simulink model "Simulink_Problema2_2"  (R2020b)
settings: Solver=VariableStepAuto  StartTime=0.0  StopTime=10.0  RelTol=1e-3
libraries: dsparch4 x2
settings Model: Creator=enrique  LastModifiedBy=enrique

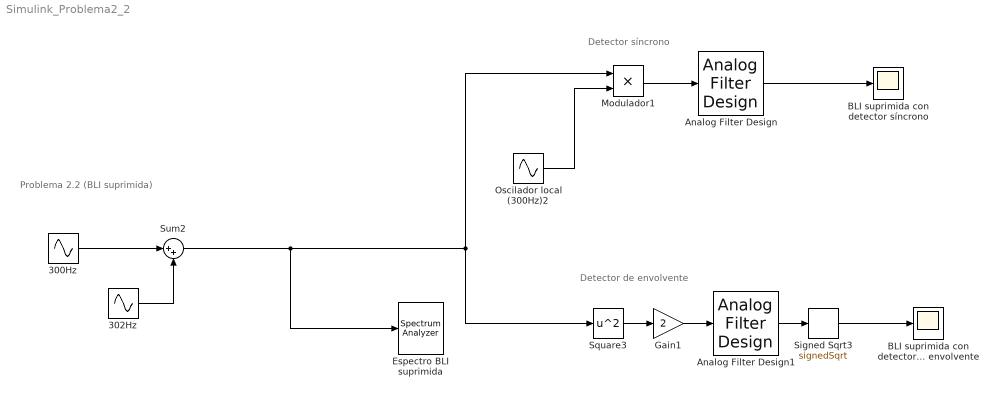
== system Simulink_Problema2_2 ==
  note: Problema 2.2 (BLI suprimida)
  note: Detector síncrono
  note: Detector de envolvente
  300Hz : Sin  Frequency=2*pi*300  SampleTime=1/5000
  302Hz : Sin  Amplitude=0.8  Frequency=2*pi*302  SampleTime=1/5000
  Analog Filter Design : dsparch4/Analog Filter Design  method=Butterworth  filttype=Lowpass  N=4  Wlo=2*pi*10  Whi=80  Rp=2  Rs=40
  Analog Filter Design1 : dsparch4/Analog Filter Design  method=Butterworth  filttype=Lowpass  N=4  Wlo=2*pi*10  Whi=80  Rp=2  Rs=40
  BLI suprimida con detector síncrono : Scope
  BLI suprimida con detector de envolvente : Scope
  Espectro BLI suprimida : SpectrumAnalyzer
  Gain1 : Gain  Gain=2
  Modulador1 : Product  OutDataTypeStr=Inherit: Same as first input
  Oscilador local (300Hz)2 : Sin  Amplitude=2  Frequency=2*pi*300  SampleTime=1/5000
  Signed Sqrt3 : Sqrt  Operator=signedSqrt  SaturateOnIntegerOverflow=on
  Square3 : Math  Operator=square  SaturateOnIntegerOverflow=on
  Sum2 : Sum  Inputs=|++
  wires:
  302Hz/1 -> Sum2/2
  300Hz/1 -> Sum2/1
  Analog Filter Design/1 -> BLI suprimida con detector síncrono/1
  Modulador1/1 -> Analog Filter Design/1
  Oscilador local (300Hz)2/1 -> Modulador1/2
  Signed Sqrt3/1 -> BLI suprimida con detector de envolvente/1
  Analog Filter Design1/1 -> Signed Sqrt3/1
  Sum2/1 -> Square3/1, Modulador1/1, Espectro BLI suprimida/1
  Square3/1 -> Gain1/1
  Gain1/1 -> Analog Filter Design1/1
